simulink model "test_pi_av_formation_event_gazebodirected23a"  (R2023a)
settings: Solver=FixedStepAuto  StartTime=0.0  StopTime=inf  RelTol=1e-3
undefined symbols (not defined in the file or in its folder): angular, DiscIntNeverNeededParam, linear
libraries: ros2lib x28, simulink x8, robotcorelib x8
(part 2 of 4)

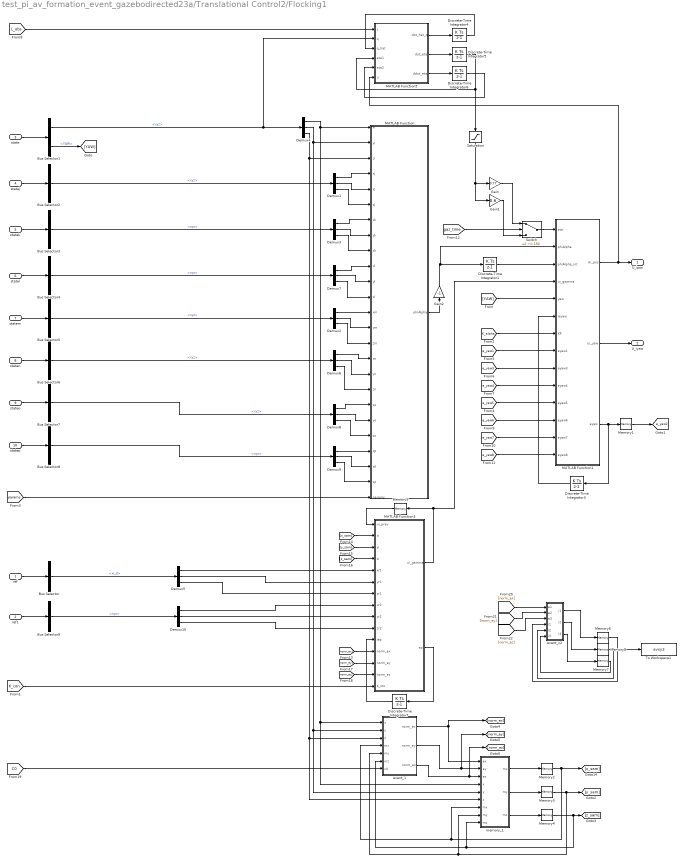
== system test_pi_av_formation_event_gazebodirected23a/Translational Control2/Flocking1 ==
  ref : Inport
  ref1 : Inport  Port=2
  state : Inport  Port=3
  statej : Inport  Port=4
  statek : Inport  Port=5
  statel : Inport  Port=6
  statem : Inport  Port=7
  staten : Inport  Port=8
  stateo : Inport  Port=9
  statep : Inport  Port=10
  Bus Selector : BusSelector  OutputSignals=xi_d
  Bus Selector1 : BusSelector  OutputSignals=xyz,YAW
  Bus Selector{2..9} (8 alike) : BusSelector  OutputSignals=xyz
  Demux{1..10} (10 alike) : Demux  Outputs=3
  Discrete-Time Integrator1 : DiscreteIntegrator  SampleTime=-1  LimitOutput=on  UpperSaturationLimit=2  LowerSaturationLimit=-2  ICPrevOutput=DiscIntNeverNeededParam  ICPrevScaledInput=DiscIntNeverNeededParam
  Discrete-Time Integrator3 : DiscreteIntegrator  SampleTime=-1  LimitOutput=on  UpperSaturationLimit=1  LowerSaturationLimit=-1  ICPrevOutput=DiscIntNeverNeededParam  ICPrevScaledInput=DiscIntNeverNeededParam
  Discrete-Time Integrator4 : DiscreteIntegrator  SampleTime=-1  LimitOutput=on  UpperSaturationLimit=5  LowerSaturationLimit=-5  ICPrevOutput=DiscIntNeverNeededParam  ICPrevScaledInput=DiscIntNeverNeededParam
  Discrete-Time Integrator5 : DiscreteIntegrator  SampleTime=-1  LimitOutput=on  UpperSaturationLimit=5  LowerSaturationLimit=-5  ICPrevOutput=DiscIntNeverNeededParam  ICPrevScaledInput=DiscIntNeverNeededParam
  Discrete-Time Integrator6 : DiscreteIntegrator  SampleTime=-1  LimitOutput=on  UpperSaturationLimit=0.2  LowerSaturationLimit=-0.2  ICPrevOutput=DiscIntNeverNeededParam  ICPrevScaledInput=DiscIntNeverNeededParam
  Discrete-Time Integrator7 : DiscreteIntegrator  SampleTime=-1  LimitOutput=on  UpperSaturationLimit=2  LowerSaturationLimit=-2  ICPrevOutput=DiscIntNeverNeededParam  ICPrevScaledInput=DiscIntNeverNeededParam
  Gain : Gain  Gain=0.77
  Gain1 : Gain  Gain=0.6
  Gain2 : Gain  Gain=-1
  MATLAB Function : MATLAB Function  TreatAsAtomicUnit=on
  MATLAB Function1 : MATLAB Function  TreatAsAtomicUnit=on
  MATLAB Function3 : MATLAB Function  TreatAsAtomicUnit=on
  MATLAB Function5 : MATLAB Function  TreatAsAtomicUnit=on
  Memory1 : Memory  InitialCondition=1
  Memory{2..4,6..8} (6 alike) : Memory
  Memory5 : Memory  InitialCondition=[0 0 0]'
  Saturation : Saturate  UpperLimit=1  LowerLimit=-1
  Switch : Switch  Threshold=150  SaturateOnIntegerOverflow=off  InputSameDT=off
  To Workspace1 : ToWorkspace  VariableName=evsy2  SampleTime=-1
  event_1 : MATLAB Function  TreatAsAtomicUnit=on
  event_x2 : MATLAB Function  TreatAsAtomicUnit=on
  memory_1 : MATLAB Function  TreatAsAtomicUnit=on
  U_ipos : Outport  VectorParamsAs1DForOutWhenUnconnected=off
  U_iyaw : Outport  Port=2  VectorParamsAs1DForOutWhenUnconnected=off
  tag scope: e_yaw2=global
  wires:
  state/1 -> Bus Selector1/1
  statej/1 -> Bus Selector2/1
  Bus Selector2/1 -> Demux1/1  "<xyz>"
  Demux1/1 -> MATLAB Function/4(xj)
  Demux1/2 -> MATLAB Function/5(yj)
  Discrete-Time Integrator1/1 -> MATLAB Function1/3(phiAlpha_int)
  statek/1 -> Bus Selector3/1
  Demux3/1 -> MATLAB Function/7(xk)
  Demux3/2 -> MATLAB Function/8(yk)
  Bus Selector3/1 -> Demux3/1  "<xyz>"
  MATLAB Function/1(phiAlpha) -> Gain2/1
  Demux3/3 -> MATLAB Function/9(zk)
  Demux1/3 -> MATLAB Function/6(zj)
  statel/1 -> Bus Selector4/1
  Demux7/1 -> MATLAB Function/10(xl)
  Demux7/2 -> MATLAB Function/11(yl)
  Demux7/3 -> MATLAB Function/12(zl)
  Bus Selector4/1 -> Demux7/1  "<xyz>"
  Bus Selector1/2 -> [YAW]  "<YAW>"
  [YAW] -> MATLAB Function1/5(yaw)
  MATLAB Function1/2(ui_yaw) -> U_iyaw/1
  MATLAB Function1/3(eyaw) -> Memory1/1, Discrete-Time Integrator3/1
  Discrete-Time Integrator3/1 -> MATLAB Function1/6(ieyaw)
  [K_alpha] -> MATLAB Function1/7(KP)
  [params] -> MATLAB Function/25(params)
  statem/1 -> Bus Selector5/1
  Bus Selector5/1 -> Demux2/1  "<xyz>"
  Demux2/1 -> MATLAB Function/13(xm)
  Demux2/2 -> MATLAB Function/14(ym)
  Demux2/3 -> MATLAB Function/15(zm)
  Memory1/1 -> [e_yaw2]
  [e_yaw1] -> MATLAB Function1/8(eyaw1)
  [e_yaw3] -> MATLAB Function1/9(eyaw3)
  [e_yaw4] -> MATLAB Function1/10(eyaw4)
  [e_yaw5] -> MATLAB Function1/11(eyaw5)
  Discrete-Time Integrator4/1 -> MATLAB Function5/3(q_hat)
  Discrete-Time Integrator5/1 -> Saturation/1, MATLAB Function5/4(eta1)
  [L_obs] -> MATLAB Function5/1(L)
  MATLAB Function5/1(dot_hat_q) -> Discrete-Time Integrator4/1
  MATLAB Function1/1(Ui_pos) -> MATLAB Function5/6(u), U_ipos/1
  Bus Selector1/1 -> MATLAB Function5/2(q), Demux4/1  "<xyz>"
  MATLAB Function5/2(dot_eta) -> Discrete-Time Integrator5/1
  Discrete-Time Integrator6/1 -> MATLAB Function5/5(eta2)
  MATLAB Function5/3(ddot_eta) -> Discrete-Time Integrator6/1
  staten/1 -> Bus Selector6/1
  Demux6/1 -> MATLAB Function/16(xn)
  Demux6/2 -> MATLAB Function/17(yn)
  Demux6/3 -> MATLAB Function/18(zn)
  Bus Selector6/1 -> Demux6/1  "<xyz>"
  [e_yaw6] -> MATLAB Function1/12(eyaw6)
  stateo/1 -> Bus Selector7/1
  Demux8/1 -> MATLAB Function/19(xo)
  Demux8/2 -> MATLAB Function/20(yo)
  Demux8/3 -> MATLAB Function/21(zo)
  Bus Selector7/1 -> Demux8/1  "<xyz>"
  [e_yaw7] -> MATLAB Function1/13(eyaw7)
  statep/1 -> Bus Selector8/1
  Demux9/1 -> MATLAB Function/22(xp)
  Demux9/2 -> MATLAB Function/23(yp)
  Demux9/3 -> MATLAB Function/24(zp)
  Bus Selector8/1 -> Demux9/1  "<xyz>"
  [e_yaw8] -> MATLAB Function1/14(eyaw8)
  Bus Selector/1 -> Demux5/1  "<xi_d>"
  Demux5/1 -> MATLAB Function3/5(xr1)
  ref/1 -> Bus Selector/1
  Demux10/1 -> MATLAB Function3/8(xr2)
  [K_con] -> MATLAB Function3/15(K_cts)
  Demux5/2 -> MATLAB Function3/6(yr1)
  ref1/1 -> Bus Selector9/1
  Demux10/3 -> MATLAB Function3/10(zr2)
  Demux10/2 -> MATLAB Function3/9(yr2)
  Demux5/3 -> MATLAB Function3/7(zr1)
  Bus Selector9/1 -> Demux10/1  "<xyz>"
  Saturation/1 -> Gain1/1, Gain/1
  Switch/1 -> MATLAB Function1/1(eta)
  [gaz_time] -> Switch/2
  Gain1/1 -> Switch/3
  Gain/1 -> Switch/1
  event_1/2(norm_ey) -> [norm_ey], memory_1/2(ey)
  Memory4/1 -> memory_1/9("mz "), event_1/6(mz), [z_sam]
  memory_1/2(my) -> Memory3/1
  memory_1/3(mz) -> Memory4/1
  Memory3/1 -> [y_sam], memory_1/8("my "), event_1/5(my)
  Demux4/1 -> event_1/1(x), memory_1/4(x), MATLAB Function/1(xi)
  event_1/3(norm_ez) -> [norm_ez], memory_1/3(ez)
  Demux4/3 -> event_1/3(z), memory_1/6(z), MATLAB Function/3(zi)
  MATLAB Function3/2(ep) -> Discrete-Time Integrator7/1
  Discrete-Time Integrator7/1 -> MATLAB Function3/11(iep)
  Demux4/2 -> event_1/2(y), memory_1/5(y), MATLAB Function/2(yi)
  event_1/1(norm_ex) -> [norm_ex], memory_1/1(ex)
  memory_1/1(mx) -> Memory2/1
  Memory2/1 -> memory_1/7("mx "), event_1/4(mx), [x_sam]
  Memory5/1 -> MATLAB Function3/1(ui_prev)
  MATLAB Function3/1(ui_gamma) -> MATLAB Function1/4(ui_gamma), Memory5/1
  [x_sam] -> MATLAB Function3/2(xi)
  [y_sam] -> MATLAB Function3/3(yi)
  [z_sam] -> MATLAB Function3/4(zi)
  [norm_ex] -> MATLAB Function3/12(norm_ex)
  [norm_ey] -> MATLAB Function3/13(norm_ey)
  [norm_ez] -> MATLAB Function3/14(norm_ez)
  [C0] -> event_1/7(c0)
  Gain2/1 -> Discrete-Time Integrator1/1, MATLAB Function1/2(phiAlpha)
  Memory7/1 -> event_x2/6("i3 ")
  [norm_ez] -> event_x2/3(e3)
  [norm_ex] -> event_x2/1(e1)
  event_x2/2(i2) -> Memory8/1
  Memory8/1 -> To Workspace1/1, event_x2/5("i2 ")
  event_x2/1(i1) -> Memory6/1
  Memory6/1 -> event_x2/4("i1 ")
  event_x2/3(i3) -> Memory7/1
  [norm_ey] -> event_x2/2(e2)

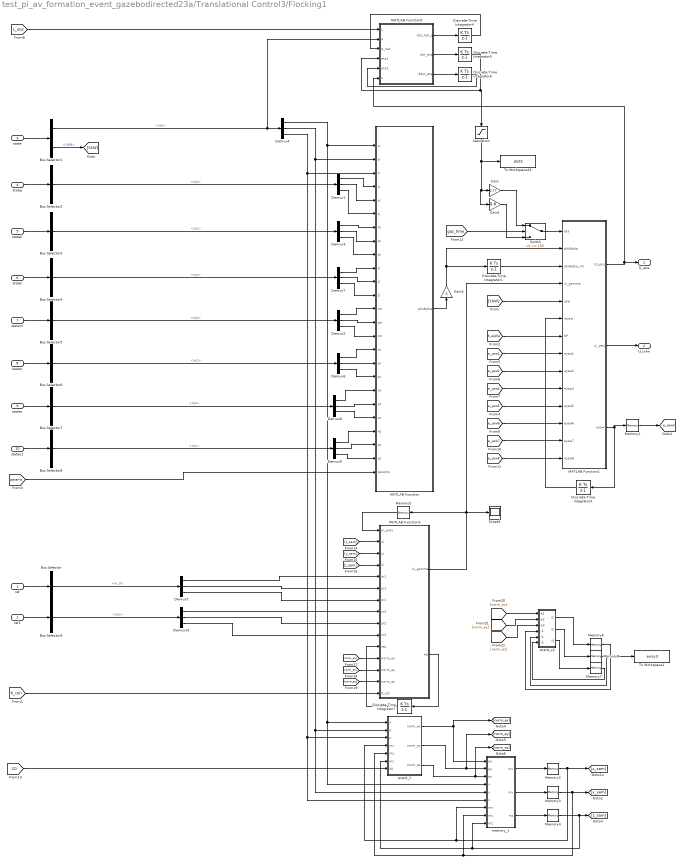
== system test_pi_av_formation_event_gazebodirected23a/Translational Control3/Flocking1 ==
  ref : Inport
  ref1 : Inport  Port=2
  state : Inport  Port=3
  statej : Inport  Port=4
  statek : Inport  Port=5
  statel : Inport  Port=6
  statem : Inport  Port=7
  staten : Inport  Port=8
  stateo : Inport  Port=9
  stateo1 : Inport  Port=10
  Bus Selector : BusSelector  OutputSignals=xi_d
  Bus Selector1 : BusSelector  OutputSignals=xyz,YAW
  Bus Selector{2..9} (8 alike) : BusSelector  OutputSignals=xyz
  Demux{1..10} (10 alike) : Demux  Outputs=3
  Discrete-Time Integrator1 : DiscreteIntegrator  SampleTime=-1  LimitOutput=on  UpperSaturationLimit=2  LowerSaturationLimit=-2  ICPrevOutput=DiscIntNeverNeededParam  ICPrevScaledInput=DiscIntNeverNeededParam
  Discrete-Time Integrator3 : DiscreteIntegrator  SampleTime=-1  LimitOutput=on  UpperSaturationLimit=1  LowerSaturationLimit=-1  ICPrevOutput=DiscIntNeverNeededParam  ICPrevScaledInput=DiscIntNeverNeededParam
  Discrete-Time Integrator4 : DiscreteIntegrator  SampleTime=-1  LimitOutput=on  UpperSaturationLimit=5  LowerSaturationLimit=-5  ICPrevOutput=DiscIntNeverNeededParam  ICPrevScaledInput=DiscIntNeverNeededParam
  Discrete-Time Integrator5 : DiscreteIntegrator  SampleTime=-1  LimitOutput=on  UpperSaturationLimit=2  LowerSaturationLimit=-2  ICPrevOutput=DiscIntNeverNeededParam  ICPrevScaledInput=DiscIntNeverNeededParam
  Discrete-Time Integrator6 : DiscreteIntegrator  SampleTime=-1  LimitOutput=on  UpperSaturationLimit=0.2  LowerSaturationLimit=-0.2  ICPrevOutput=DiscIntNeverNeededParam  ICPrevScaledInput=DiscIntNeverNeededParam
  Discrete-Time Integrator7 : DiscreteIntegrator  SampleTime=-1  LimitOutput=on  UpperSaturationLimit=2  LowerSaturationLimit=-2  ICPrevOutput=DiscIntNeverNeededParam  ICPrevScaledInput=DiscIntNeverNeededParam
  Gain : Gain  Gain=0.77
  Gain1 : Gain  Gain=0.6
  Gain2 : Gain  Gain=-1
  MATLAB Function : MATLAB Function  TreatAsAtomicUnit=on
  MATLAB Function1 : MATLAB Function  TreatAsAtomicUnit=on
  MATLAB Function3 : MATLAB Function  TreatAsAtomicUnit=on
  MATLAB Function5 : MATLAB Function  TreatAsAtomicUnit=on
  Memory1 : Memory  InitialCondition=1
  Memory{2..4,6..8} (6 alike) : Memory
  Memory5 : Memory  InitialCondition=[0 0 0]'
  Saturation : Saturate  UpperLimit=1  LowerLimit=-1
  Scope1 : Scope
  Switch : Switch  Threshold=150  SaturateOnIntegerOverflow=off  InputSameDT=off
  To Workspace1 : ToWorkspace  VariableName=evsy3  SampleTime=-1
  To Workspace24 : ToWorkspace  VariableName=dist3  SampleTime=-1
  event_1 : MATLAB Function  TreatAsAtomicUnit=on
  event_x2 : MATLAB Function  TreatAsAtomicUnit=on
  memory_1 : MATLAB Function  TreatAsAtomicUnit=on
  U_ipos : Outport  VectorParamsAs1DForOutWhenUnconnected=off
  U_iyaw : Outport  Port=2  VectorParamsAs1DForOutWhenUnconnected=off
  tag scope: e_yaw3=global
  wires:
  state/1 -> Bus Selector1/1
  statej/1 -> Bus Selector2/1
  Bus Selector2/1 -> Demux1/1  "<xyz>"
  Demux1/1 -> MATLAB Function/4(xj)
  Demux1/2 -> MATLAB Function/5(yj)
  Discrete-Time Integrator1/1 -> MATLAB Function1/3(phiAlpha_int)
  statek/1 -> Bus Selector3/1
  Demux3/1 -> MATLAB Function/7(xk)
  Demux3/2 -> MATLAB Function/8(yk)
  Bus Selector3/1 -> Demux3/1  "<xyz>"
  MATLAB Function/1(phiAlpha) -> Gain2/1
  Demux3/3 -> MATLAB Function/9(zk)
  Demux1/3 -> MATLAB Function/6(zj)
  statel/1 -> Bus Selector4/1
  Demux7/1 -> MATLAB Function/10(xl)
  Demux7/2 -> MATLAB Function/11(yl)
  Demux7/3 -> MATLAB Function/12(zl)
  Bus Selector4/1 -> Demux7/1  "<xyz>"
  Bus Selector1/2 -> [YAW]  "<YAW>"
  [YAW] -> MATLAB Function1/5(yaw)
  MATLAB Function1/2(ui_yaw) -> U_iyaw/1
  MATLAB Function1/3(eyaw) -> Memory1/1, Discrete-Time Integrator3/1
  Discrete-Time Integrator3/1 -> MATLAB Function1/6(ieyaw)
  [K_alpha] -> MATLAB Function1/7(KP)
  [params] -> MATLAB Function/25(params)
  statem/1 -> Bus Selector5/1
  Bus Selector5/1 -> Demux2/1  "<xyz>"
  Demux2/1 -> MATLAB Function/13(xm)
  Demux2/2 -> MATLAB Function/14(ym)
  Demux2/3 -> MATLAB Function/15(zm)
  Memory1/1 -> [e_yaw3]
  [e_yaw1] -> MATLAB Function1/8(eyaw1)
  [e_yaw2] -> MATLAB Function1/9(eyaw2)
  [e_yaw4] -> MATLAB Function1/10(eyaw4)
  [e_yaw5] -> MATLAB Function1/11(eyaw5)
  Discrete-Time Integrator4/1 -> MATLAB Function5/3(q_hat)
  Discrete-Time Integrator5/1 -> Saturation/1, MATLAB Function5/4(eta1)
  [L_obs] -> MATLAB Function5/1(L)
  MATLAB Function5/1(dot_hat_q) -> Discrete-Time Integrator4/1
  MATLAB Function1/1(Ui_pos) -> MATLAB Function5/6(u), U_ipos/1
  Bus Selector1/1 -> MATLAB Function5/2(q), Demux4/1  "<xyz>"
  MATLAB Function5/2(dot_eta) -> Discrete-Time Integrator5/1
  Discrete-Time Integrator6/1 -> MATLAB Function5/5(eta2)
  MATLAB Function5/3(ddot_eta) -> Discrete-Time Integrator6/1
  staten/1 -> Bus Selector6/1
  Demux6/1 -> MATLAB Function/16(xn)
  Demux6/2 -> MATLAB Function/17(yn)
  Demux6/3 -> MATLAB Function/18(zn)
  Bus Selector6/1 -> Demux6/1  "<xyz>"
  [e_yaw6] -> MATLAB Function1/12(eyaw6)
  [e_yaw7] -> MATLAB Function1/13(eyaw7)
  stateo/1 -> Bus Selector7/1
  Demux8/1 -> MATLAB Function/19(xo)
  Demux8/2 -> MATLAB Function/20(yo)
  Demux8/3 -> MATLAB Function/21(zo)
  Bus Selector7/1 -> Demux8/1  "<xyz>"
  stateo1/1 -> Bus Selector8/1
  Demux9/1 -> MATLAB Function/22(xp)
  Demux9/2 -> MATLAB Function/23(yp)
  Demux9/3 -> MATLAB Function/24(zp)
  Bus Selector8/1 -> Demux9/1  "<xyz>"
  [e_yaw8] -> MATLAB Function1/14(eyaw8)
  Bus Selector/1 -> Demux5/1  "<xi_d>"
  ref/1 -> Bus Selector/1
  ref1/1 -> Bus Selector9/1
  Bus Selector9/1 -> Demux10/1  "<xyz>"
  Switch/1 -> MATLAB Function1/1(eta)
  [gaz_time] -> Switch/2
  Gain1/1 -> Switch/3
  Gain/1 -> Switch/1
  Saturation/1 -> To Workspace24/1, Gain1/1, Gain/1
  Memory4/1 -> memory_1/9("mz "), event_1/6(mz), [z_sam]
  memory_1/2(my) -> Memory3/1
  memory_1/3(mz) -> Memory4/1
  Memory3/1 -> [y_sam], memory_1/8("my "), event_1/5(my)
  Demux4/1 -> memory_1/4(x), event_1/1(x), MATLAB Function/1(xi)
  event_1/3(norm_ez) -> [norm_ez], memory_1/3(ez)
  event_1/1(norm_ex) -> [norm_ex], memory_1/1(ex)
  MATLAB Function3/1(ui_gamma) -> MATLAB Function1/4(ui_gamma), Scope1/1, Memory5/1
  event_1/2(norm_ey) -> [norm_ey], memory_1/2(ey)
  Demux4/3 -> memory_1/6(z), event_1/3(z), MATLAB Function/3(zi)
  MATLAB Function3/2(ep) -> Discrete-Time Integrator7/1
  memory_1/1(mx) -> Memory2/1
  Discrete-Time Integrator7/1 -> MATLAB Function3/11(iep)
  Demux4/2 -> memory_1/5(y), event_1/2(y), MATLAB Function/2(yi)
  Memory2/1 -> memory_1/7("mx "), event_1/4(mx), [x_sam]
  Memory5/1 -> MATLAB Function3/1(ui_prev)
  [K_con] -> MATLAB Function3/15(K_cts)
  Demux5/1 -> MATLAB Function3/5(xr1)
  Demux5/2 -> MATLAB Function3/6(yr1)
  Demux5/3 -> MATLAB Function3/7(zr1)
  Demux10/1 -> MATLAB Function3/8(xr2)
  Demux10/2 -> MATLAB Function3/9(yr2)
  Demux10/3 -> MATLAB Function3/10(zr2)
  [y_sam] -> MATLAB Function3/3(yi)
  [x_sam] -> MATLAB Function3/2(xi)
  [z_sam] -> MATLAB Function3/4(zi)
  [norm_ez] -> MATLAB Function3/14(norm_ez)
  [norm_ey] -> MATLAB Function3/13(norm_ey)
  [norm_ex] -> MATLAB Function3/12(norm_ex)
  [C0] -> event_1/7(c0)
  Gain2/1 -> MATLAB Function1/2(phiAlpha), Discrete-Time Integrator1/1
  Memory7/1 -> event_x2/6("i3 ")
  [norm_ez] -> event_x2/3(e3)
  [norm_ex] -> event_x2/1(e1)
  event_x2/2(i2) -> Memory8/1
  Memory8/1 -> To Workspace1/1, event_x2/5("i2 ")
  event_x2/1(i1) -> Memory6/1
  Memory6/1 -> event_x2/4("i1 ")
  event_x2/3(i3) -> Memory7/1
  [norm_ey] -> event_x2/2(e2)

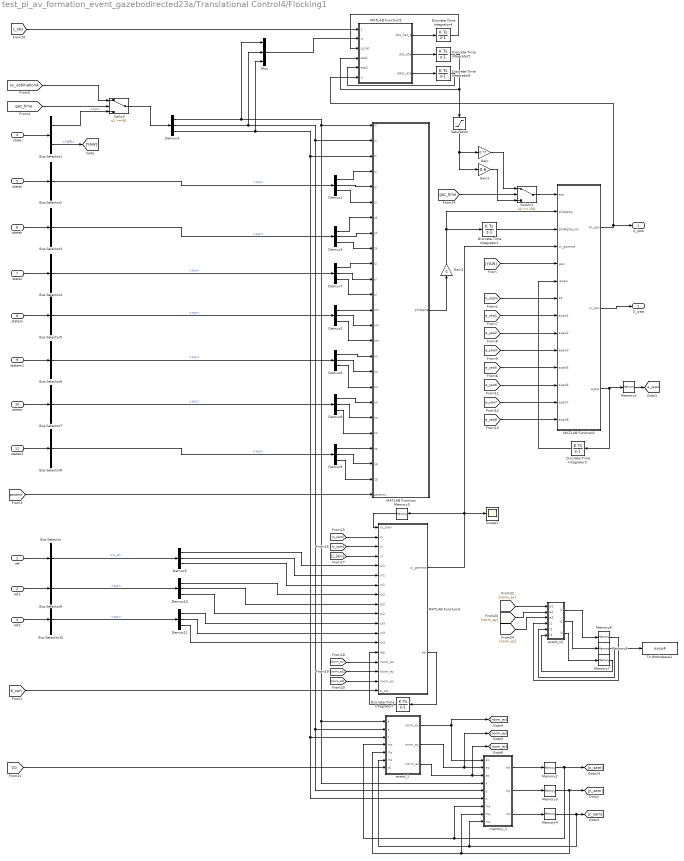
== system test_pi_av_formation_event_gazebodirected23a/Translational Control4/Flocking1 ==
  ref : Inport
  ref1 : Inport  Port=2
  ref2 : Inport  Port=3
  state : Inport  Port=4
  statej : Inport  Port=5
  statek : Inport  Port=6
  statel : Inport  Port=7
  statem : Inport  Port=8
  statem1 : Inport  Port=9
  stateo : Inport  Port=10
  stateo1 : Inport  Port=11
  Bus Selector : BusSelector  OutputSignals=xi_d
  Bus Selector1 : BusSelector  OutputSignals=xyz,YAW
  Bus Selector{2..10} (9 alike) : BusSelector  OutputSignals=xyz
  Demux{1..11} (11 alike) : Demux  Outputs=3
  Discrete-Time Integrator1 : DiscreteIntegrator  SampleTime=-1  LimitOutput=on  UpperSaturationLimit=2  LowerSaturationLimit=-2  ICPrevOutput=DiscIntNeverNeededParam  ICPrevScaledInput=DiscIntNeverNeededParam
  Discrete-Time Integrator3 : DiscreteIntegrator  SampleTime=-1  LimitOutput=on  UpperSaturationLimit=1  LowerSaturationLimit=-1  ICPrevOutput=DiscIntNeverNeededParam  ICPrevScaledInput=DiscIntNeverNeededParam
  Discrete-Time Integrator4 : DiscreteIntegrator  SampleTime=-1  LimitOutput=on  UpperSaturationLimit=5  LowerSaturationLimit=-5  ICPrevOutput=DiscIntNeverNeededParam  ICPrevScaledInput=DiscIntNeverNeededParam
  Discrete-Time Integrator5 : DiscreteIntegrator  SampleTime=-1  LimitOutput=on  UpperSaturationLimit=5  LowerSaturationLimit=-5  ICPrevOutput=DiscIntNeverNeededParam  ICPrevScaledInput=DiscIntNeverNeededParam
  Discrete-Time Integrator6 : DiscreteIntegrator  SampleTime=-1  LimitOutput=on  UpperSaturationLimit=0.2  LowerSaturationLimit=-0.2  ICPrevOutput=DiscIntNeverNeededParam  ICPrevScaledInput=DiscIntNeverNeededParam
  Discrete-Time Integrator7 : DiscreteIntegrator  SampleTime=-1  LimitOutput=on  UpperSaturationLimit=2  LowerSaturationLimit=-2  ICPrevOutput=DiscIntNeverNeededParam  ICPrevScaledInput=DiscIntNeverNeededParam
  Gain : Gain  Gain=0.77
  Gain1 : Gain  Gain=0.6
  Gain2 : Gain  Gain=-1
  MATLAB Function : MATLAB Function  TreatAsAtomicUnit=on
  MATLAB Function1 : MATLAB Function  TreatAsAtomicUnit=on
  MATLAB Function3 : MATLAB Function  TreatAsAtomicUnit=on
  MATLAB Function5 : MATLAB Function  TreatAsAtomicUnit=on
  Memory1 : Memory  InitialCondition=1
  Memory{2..4,6..8} (6 alike) : Memory
  Memory5 : Memory  InitialCondition=[0 0 0]'
  Mux : Mux  Inputs=3
  Saturation : Saturate  UpperLimit=1  LowerLimit=-1
  Scope1 : Scope
  Switch : Switch  Threshold=60  SaturateOnIntegerOverflow=off  InputSameDT=off
  Switch1 : Switch  Threshold=150  SaturateOnIntegerOverflow=off  InputSameDT=off
  To Workspace1 : ToWorkspace  VariableName=evsy4  SampleTime=-1
  event_1 : MATLAB Function  TreatAsAtomicUnit=on
  event_x2 : MATLAB Function  TreatAsAtomicUnit=on
  memory_1 : MATLAB Function  TreatAsAtomicUnit=on
  U_ipos : Outport  VectorParamsAs1DForOutWhenUnconnected=off
  U_iyaw : Outport  Port=2  VectorParamsAs1DForOutWhenUnconnected=off
  tag scope: e_yaw4=global
  wires:
  ref/1 -> Bus Selector/1
  state/1 -> Bus Selector1/1
  Bus Selector/1 -> Demux5/1  "<xi_d>"
  statej/1 -> Bus Selector2/1
  Bus Selector2/1 -> Demux1/1  "<xyz>"
  Demux1/1 -> MATLAB Function/4(xj)
  Demux1/2 -> MATLAB Function/5(yj)
  Discrete-Time Integrator1/1 -> MATLAB Function1/3(phiAlpha_int)
  statek/1 -> Bus Selector3/1
  Demux3/1 -> MATLAB Function/7(xk)
  Demux3/2 -> MATLAB Function/8(yk)
  Bus Selector3/1 -> Demux3/1  "<xyz>"
  MATLAB Function/1(phiAlpha) -> Gain2/1
  Demux3/3 -> MATLAB Function/9(zk)
  Demux1/3 -> MATLAB Function/6(zj)
  statel/1 -> Bus Selector4/1
  Demux7/1 -> MATLAB Function/10(xl)
  Demux7/2 -> MATLAB Function/11(yl)
  Demux7/3 -> MATLAB Function/12(zl)
  Bus Selector4/1 -> Demux7/1  "<xyz>"
  Bus Selector1/2 -> [YAW]  "<YAW>"
  [YAW] -> MATLAB Function1/5(yaw)
  MATLAB Function1/2(ui_yaw) -> U_iyaw/1
  [K_con] -> MATLAB Function3/18(K_cts)
  MATLAB Function1/3(eyaw) -> Memory1/1, Discrete-Time Integrator3/1
  Discrete-Time Integrator3/1 -> MATLAB Function1/6(ieyaw)
  [K_alpha] -> MATLAB Function1/7(KP)
  [params] -> MATLAB Function/25(params)
  statem/1 -> Bus Selector5/1
  Bus Selector5/1 -> Demux2/1  "<xyz>"
  Demux2/1 -> MATLAB Function/13(xm)
  Demux2/2 -> MATLAB Function/14(ym)
  Demux2/3 -> MATLAB Function/15(zm)
  [gaz_time] -> Switch/2
  [xy_estimation4] -> Switch/1
  [e_yaw1] -> MATLAB Function1/8(eyaw1)
  [e_yaw2] -> MATLAB Function1/9(eyaw2)
  [e_yaw3] -> MATLAB Function1/10(eyaw3)
  [e_yaw5] -> MATLAB Function1/11(eyaw5)
  Memory1/1 -> [e_yaw4]
  Mux/1 -> MATLAB Function5/2(q)
  MATLAB Function5/1(dot_hat_q) -> Discrete-Time Integrator4/1
  Discrete-Time Integrator6/1 -> MATLAB Function5/5(eta2)
  MATLAB Function5/3(ddot_eta) -> Discrete-Time Integrator6/1
  Discrete-Time Integrator5/1 -> Saturation/1, MATLAB Function5/4(eta1)
  MATLAB Function5/2(dot_eta) -> Discrete-Time Integrator5/1
  Discrete-Time Integrator4/1 -> MATLAB Function5/3(q_hat)
  [L_obs] -> MATLAB Function5/1(L)
  MATLAB Function1/1(Ui_pos) -> MATLAB Function5/6(u), U_ipos/1
  statem1/1 -> Bus Selector6/1
  Demux6/1 -> MATLAB Function/16(xn)
  Demux6/2 -> MATLAB Function/17(yn)
  Demux6/3 -> MATLAB Function/18(zn)
  Bus Selector6/1 -> Demux6/1  "<xyz>"
  Bus Selector1/1 -> Switch/3  "<xyz>"
  Switch/1 -> Demux4/1
  stateo/1 -> Bus Selector7/1
  Demux8/1 -> MATLAB Function/19(xo)
  Demux8/2 -> MATLAB Function/20(yo)
  Demux8/3 -> MATLAB Function/21(zo)
  Bus Selector7/1 -> Demux8/1  "<xyz>"
  [e_yaw6] -> MATLAB Function1/12(eyaw6)
  [e_yaw7] -> MATLAB Function1/13(eyaw7)
  stateo1/1 -> Bus Selector8/1
  Demux9/1 -> MATLAB Function/22(xp)
  Demux9/2 -> MATLAB Function/23(yp)
  Demux9/3 -> MATLAB Function/24(zp)
  Bus Selector8/1 -> Demux9/1  "<xyz>"
  [e_yaw8] -> MATLAB Function1/14(eyaw8)
  Bus Selector9/1 -> Demux10/1  "<xyz>"
  ref1/1 -> Bus Selector9/1
  Switch1/1 -> MATLAB Function1/1(eta)
  Gain/1 -> Switch1/1
  Gain1/1 -> Switch1/3
  [gaz_time] -> Switch1/2
  Saturation/1 -> Gain1/1, Gain/1
  ref2/1 -> Bus Selector10/1
  Bus Selector10/1 -> Demux11/1  "<xyz>"
  event_1/2(norm_ey) -> [norm_ey], memory_1/2(ey)
  MATLAB Function3/1(ui_gamma) -> MATLAB Function1/4(ui_gamma), Scope1/1, Memory5/1
  Memory4/1 -> memory_1/9("mz "), event_1/6(mz), [z_sam]
  memory_1/2(my) -> Memory3/1
  memory_1/3(mz) -> Memory4/1
  Memory3/1 -> [y_sam], memory_1/8("my "), event_1/5(my)
  Demux4/1 -> Mux/1, event_1/1(x), memory_1/4(x), MATLAB Function/1(xi)
  event_1/3(norm_ez) -> [norm_ez], memory_1/3(ez)
  Demux4/3 -> Mux/3, event_1/3(z), memory_1/6(z), MATLAB Function/3(zi)
  MATLAB Function3/2(ep) -> Discrete-Time Integrator7/1
  memory_1/1(mx) -> Memory2/1
  Discrete-Time Integrator7/1 -> MATLAB Function3/14(iep)
  Demux4/2 -> Mux/2, event_1/2(y), memory_1/5(y), MATLAB Function/2(yi)
  event_1/1(norm_ex) -> [norm_ex], memory_1/1(ex)
  Memory2/1 -> memory_1/7("mx "), event_1/4(mx), [x_sam]
  Memory5/1 -> MATLAB Function3/1(ui_prev)
  [x_sam] -> MATLAB Function3/2(xi)
  [y_sam] -> MATLAB Function3/3(yi)
  [z_sam] -> MATLAB Function3/4(zi)
  [norm_ex] -> MATLAB Function3/15(norm_ex)
  [norm_ey] -> MATLAB Function3/16(norm_ey)
  [norm_ez] -> MATLAB Function3/17(norm_ez)
  Demux5/1 -> MATLAB Function3/5(xr1)
  Demux5/2 -> MATLAB Function3/6(yr1)
  Demux5/3 -> MATLAB Function3/7(zr1)
  Demux10/1 -> MATLAB Function3/8(xr2)
  Demux10/2 -> MATLAB Function3/9(yr2)
  Demux10/3 -> MATLAB Function3/10(zr2)
  Demux11/1 -> MATLAB Function3/11(xr3)
  Demux11/2 -> MATLAB Function3/12(yr3)
  Demux11/3 -> MATLAB Function3/13(zr3)
  [C0] -> event_1/7(c0)
  Gain2/1 -> MATLAB Function1/2(phiAlpha), Discrete-Time Integrator1/1
  Memory7/1 -> event_x2/6("i3 ")
  [norm_ez] -> event_x2/3(e3)
  [norm_ex] -> event_x2/1(e1)
  event_x2/2(i2) -> Memory8/1
  Memory8/1 -> To Workspace1/1, event_x2/5("i2 ")
  event_x2/1(i1) -> Memory6/1
  Memory6/1 -> event_x2/4("i1 ")
  event_x2/3(i3) -> Memory7/1
  [norm_ey] -> event_x2/2(e2)

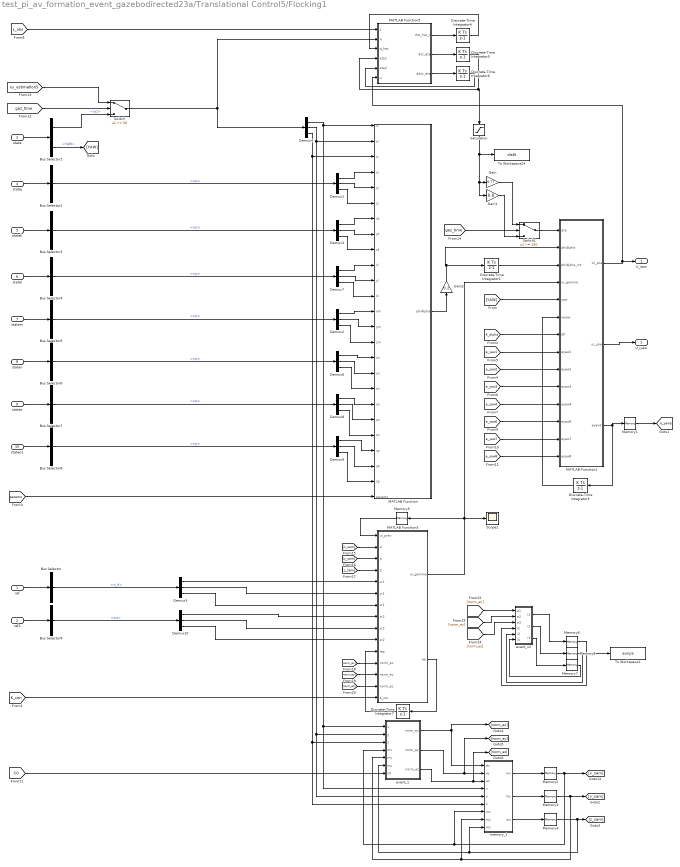
== system test_pi_av_formation_event_gazebodirected23a/Translational Control5/Flocking1 ==
  ref : Inport
  ref1 : Inport  Port=2
  state : Inport  Port=3
  statej : Inport  Port=4
  statek : Inport  Port=5
  statel : Inport  Port=6
  statem : Inport  Port=7
  staten : Inport  Port=8
  stateo : Inport  Port=9
  stateo1 : Inport  Port=10
  Bus Selector : BusSelector  OutputSignals=xi_d
  Bus Selector1 : BusSelector  OutputSignals=xyz,YAW
  Bus Selector{2..9} (8 alike) : BusSelector  OutputSignals=xyz
  Demux{1..10} (10 alike) : Demux  Outputs=3
  Discrete-Time Integrator1 : DiscreteIntegrator  SampleTime=-1  LimitOutput=on  UpperSaturationLimit=2  LowerSaturationLimit=-2  ICPrevOutput=DiscIntNeverNeededParam  ICPrevScaledInput=DiscIntNeverNeededParam
  Discrete-Time Integrator3 : DiscreteIntegrator  SampleTime=-1  LimitOutput=on  UpperSaturationLimit=1  LowerSaturationLimit=-1  ICPrevOutput=DiscIntNeverNeededParam  ICPrevScaledInput=DiscIntNeverNeededParam
  Discrete-Time Integrator4 : DiscreteIntegrator  SampleTime=-1  LimitOutput=on  UpperSaturationLimit=5  LowerSaturationLimit=-5  ICPrevOutput=DiscIntNeverNeededParam  ICPrevScaledInput=DiscIntNeverNeededParam
  Discrete-Time Integrator5 : DiscreteIntegrator  SampleTime=-1  LimitOutput=on  UpperSaturationLimit=5  LowerSaturationLimit=-5  ICPrevOutput=DiscIntNeverNeededParam  ICPrevScaledInput=DiscIntNeverNeededParam
  Discrete-Time Integrator6 : DiscreteIntegrator  SampleTime=-1  LimitOutput=on  UpperSaturationLimit=0.4  LowerSaturationLimit=-0.4  ICPrevOutput=DiscIntNeverNeededParam  ICPrevScaledInput=DiscIntNeverNeededParam
  Discrete-Time Integrator7 : DiscreteIntegrator  SampleTime=-1  LimitOutput=on  UpperSaturationLimit=2  LowerSaturationLimit=-2  ICPrevOutput=DiscIntNeverNeededParam  ICPrevScaledInput=DiscIntNeverNeededParam
  Gain : Gain  Gain=0.77
  Gain1 : Gain  Gain=0.6
  Gain2 : Gain  Gain=0.2
  MATLAB Function : MATLAB Function  TreatAsAtomicUnit=on
  MATLAB Function1 : MATLAB Function  TreatAsAtomicUnit=on
  MATLAB Function3 : MATLAB Function  TreatAsAtomicUnit=on
  MATLAB Function5 : MATLAB Function  TreatAsAtomicUnit=on
  Memory1 : Memory  InitialCondition=1
  Memory{2..4,6..8} (6 alike) : Memory
  Memory5 : Memory  InitialCondition=[0 0 0]'
  Saturation : Saturate  UpperLimit=1  LowerLimit=-1
  Scope1 : Scope
  Switch : Switch  Threshold=50  SaturateOnIntegerOverflow=off  InputSameDT=off
  Switch1 : Switch  Threshold=150  SaturateOnIntegerOverflow=off  InputSameDT=off
  To Workspace1 : ToWorkspace  VariableName=evsy5  SampleTime=-1
  To Workspace24 : ToWorkspace  VariableName=dist5  SampleTime=-1
  event_1 : MATLAB Function  TreatAsAtomicUnit=on
  event_x2 : MATLAB Function  TreatAsAtomicUnit=on
  memory_1 : MATLAB Function  TreatAsAtomicUnit=on
  U_ipos : Outport  VectorParamsAs1DForOutWhenUnconnected=off
  U_iyaw : Outport  Port=2  VectorParamsAs1DForOutWhenUnconnected=off
  tag scope: e_yaw5=global
  wires:
  ref/1 -> Bus Selector/1
  state/1 -> Bus Selector1/1
  Bus Selector/1 -> Demux5/1  "<xi_d>"
  statej/1 -> Bus Selector2/1
  Bus Selector2/1 -> Demux1/1  "<xyz>"
  Demux1/1 -> MATLAB Function/4(xj)
  Demux1/2 -> MATLAB Function/5(yj)
  Discrete-Time Integrator1/1 -> MATLAB Function1/3(phiAlpha_int)
  statek/1 -> Bus Selector3/1
  Demux3/1 -> MATLAB Function/7(xk)
  Demux3/2 -> MATLAB Function/8(yk)
  Bus Selector3/1 -> Demux3/1  "<xyz>"
  MATLAB Function/1(phiAlpha) -> Gain2/1
  Demux3/3 -> MATLAB Function/9(zk)
  Demux1/3 -> MATLAB Function/6(zj)
  statel/1 -> Bus Selector4/1
  Demux7/1 -> MATLAB Function/10(xl)
  Demux7/2 -> MATLAB Function/11(yl)
  Demux7/3 -> MATLAB Function/12(zl)
  Bus Selector4/1 -> Demux7/1  "<xyz>"
  Bus Selector1/2 -> [YAW]  "<YAW>"
  [YAW] -> MATLAB Function1/5(yaw)
  MATLAB Function1/2(ui_yaw) -> U_iyaw/1
  MATLAB Function1/3(eyaw2) -> Memory1/1, Discrete-Time Integrator3/1
  Discrete-Time Integrator3/1 -> MATLAB Function1/6(ieyaw)
  [K_alpha] -> MATLAB Function1/7(KP)
  [params] -> MATLAB Function/25(params)
  statem/1 -> Bus Selector5/1
  Bus Selector5/1 -> Demux2/1  "<xyz>"
  Demux2/1 -> MATLAB Function/13(xm)
  Demux2/2 -> MATLAB Function/14(ym)
  Demux2/3 -> MATLAB Function/15(zm)
  Memory1/1 -> [e_yaw5]
  [e_yaw1] -> MATLAB Function1/8(eyaw1)
  [e_yaw3] -> MATLAB Function1/10(eyaw3)
  [e_yaw4] -> MATLAB Function1/11(eyaw4)
  [e_yaw2] -> MATLAB Function1/9("eyaw2 ")
  Discrete-Time Integrator4/1 -> MATLAB Function5/3(q_hat)
  Discrete-Time Integrator5/1 -> Saturation/1, MATLAB Function5/4(eta1)
  [L_obs] -> MATLAB Function5/1(L)
  MATLAB Function5/1(dot_hat_q) -> Discrete-Time Integrator4/1
  MATLAB Function1/1(Ui_pos) -> MATLAB Function5/6(u), U_ipos/1
  MATLAB Function5/2(dot_eta) -> Discrete-Time Integrator5/1
  Discrete-Time Integrator6/1 -> MATLAB Function5/5(eta2)
  MATLAB Function5/3(ddot_eta) -> Discrete-Time Integrator6/1
  staten/1 -> Bus Selector6/1
  Demux6/1 -> MATLAB Function/16(xn)
  Demux6/2 -> MATLAB Function/17(yn)
  Demux6/3 -> MATLAB Function/18(zn)
  Bus Selector6/1 -> Demux6/1  "<xyz>"
  [e_yaw6] -> MATLAB Function1/12(eyaw6)
  stateo/1 -> Bus Selector7/1
  Demux8/1 -> MATLAB Function/19(xo)
  Demux8/2 -> MATLAB Function/20(yo)
  Demux8/3 -> MATLAB Function/21(zo)
  Bus Selector7/1 -> Demux8/1  "<xyz>"
  [e_yaw7] -> MATLAB Function1/13(eyaw7)
  stateo1/1 -> Bus Selector8/1
  Demux9/1 -> MATLAB Function/22(xp)
  Demux9/2 -> MATLAB Function/23(yp)
  Demux9/3 -> MATLAB Function/24(zp)
  Bus Selector8/1 -> Demux9/1  "<xyz>"
  [e_yaw8] -> MATLAB Function1/14(eyaw8)
  Switch/1 -> MATLAB Function5/2(q), Demux4/1
  Bus Selector1/1 -> Switch/3  "<xyz>"
  [xy_estimation5] -> Switch/1
  [gaz_time] -> Switch/2
  Bus Selector9/1 -> Demux10/1  "<xyz>"
  ref1/1 -> Bus Selector9/1
  Saturation/1 -> To Workspace24/1, Gain1/1, Gain/1
  Switch1/1 -> MATLAB Function1/1(eta)
  Gain1/1 -> Switch1/3
  Gain/1 -> Switch1/1
  [gaz_time] -> Switch1/2
  MATLAB Function3/1(ui_gamma) -> MATLAB Function1/4(ui_gamma), Scope1/1, Memory5/1
  event_1/1(norm_ex) -> [norm_ex], memory_1/1(ex)
  Demux4/1 -> memory_1/4(x), event_1/1(x), MATLAB Function/1(xi)
  event_1/3(norm_ez) -> [norm_ez], memory_1/3(ez)
  Demux4/2 -> memory_1/5(y), event_1/2(y), MATLAB Function/2(yi)
  Demux4/3 -> memory_1/6(z), event_1/3(z), MATLAB Function/3(zi)
  Memory4/1 -> memory_1/9("mz "), event_1/6(mz), [z_sam]
  Memory2/1 -> memory_1/7("mx "), event_1/4(mx), [x_sam]
  [y_sam] -> MATLAB Function3/3(yi)
  memory_1/3(mz) -> Memory4/1
  Memory5/1 -> MATLAB Function3/1(ui_prev)
  Memory3/1 -> [y_sam], memory_1/8("my "), event_1/5(my)
  [norm_ey] -> MATLAB Function3/13(norm_ey)
  [x_sam] -> MATLAB Function3/2(xi)
  event_1/2(norm_ey) -> [norm_ey], memory_1/2(ey)
  MATLAB Function3/2(ep) -> Discrete-Time Integrator7/1
  memory_1/1(mx) -> Memory2/1
  Discrete-Time Integrator7/1 -> MATLAB Function3/11(iep)
  [z_sam] -> MATLAB Function3/4(zi)
  memory_1/2(my) -> Memory3/1
  [norm_ez] -> MATLAB Function3/14(norm_ez)
  [norm_ex] -> MATLAB Function3/12(norm_ex)
  Demux5/1 -> MATLAB Function3/5(xr1)
  Demux5/2 -> MATLAB Function3/6(yr1)
  Demux5/3 -> MATLAB Function3/7(zr1)
  Demux10/1 -> MATLAB Function3/8(xr2)
  Demux10/2 -> MATLAB Function3/9(yr2)
  Demux10/3 -> MATLAB Function3/10(zr2)
  [K_con] -> MATLAB Function3/15(K_cts)
  [C0] -> event_1/7(c0)
  Gain2/1 -> MATLAB Function1/2(phiAlpha), Discrete-Time Integrator1/1
  Memory7/1 -> event_x2/6("i3 ")
  [norm_ez] -> event_x2/3(e3)
  [norm_ex] -> event_x2/1(e1)
  event_x2/2(i2) -> Memory8/1
  Memory8/1 -> To Workspace1/1, event_x2/5("i2 ")
  event_x2/1(i1) -> Memory6/1
  Memory6/1 -> event_x2/4("i1 ")
  event_x2/3(i3) -> Memory7/1
  [norm_ey] -> event_x2/2(e2)

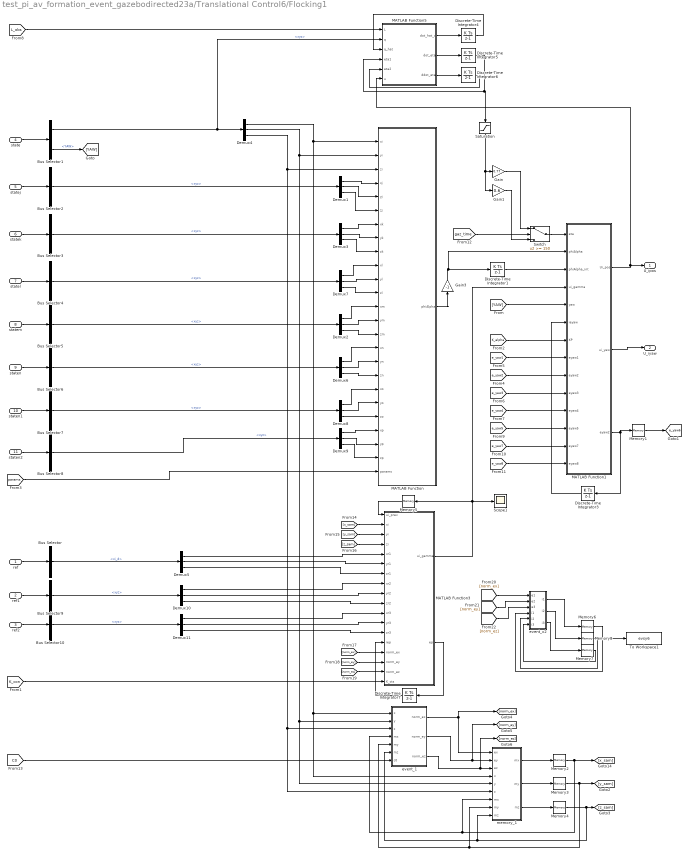
== system test_pi_av_formation_event_gazebodirected23a/Translational Control6/Flocking1 ==
  ref : Inport
  ref1 : Inport  Port=2
  ref2 : Inport  Port=3
  state : Inport  Port=4
  statej : Inport  Port=5
  statek : Inport  Port=6
  statel : Inport  Port=7
  statem : Inport  Port=8
  staten : Inport  Port=9
  staten1 : Inport  Port=10
  staten2 : Inport  Port=11
  Bus Selector : BusSelector  OutputSignals=xi_d
  Bus Selector1 : BusSelector  OutputSignals=xyz,YAW
  Bus Selector{2..10} (9 alike) : BusSelector  OutputSignals=xyz
  Demux{1..11} (11 alike) : Demux  Outputs=3
  Discrete-Time Integrator1 : DiscreteIntegrator  SampleTime=-1  LimitOutput=on  UpperSaturationLimit=2  LowerSaturationLimit=-2  ICPrevOutput=DiscIntNeverNeededParam  ICPrevScaledInput=DiscIntNeverNeededParam
  Discrete-Time Integrator3 : DiscreteIntegrator  SampleTime=-1  LimitOutput=on  UpperSaturationLimit=1  LowerSaturationLimit=-1  ICPrevOutput=DiscIntNeverNeededParam  ICPrevScaledInput=DiscIntNeverNeededParam
  Discrete-Time Integrator4 : DiscreteIntegrator  SampleTime=-1  LimitOutput=on  UpperSaturationLimit=5  LowerSaturationLimit=-5  ICPrevOutput=DiscIntNeverNeededParam  ICPrevScaledInput=DiscIntNeverNeededParam
  Discrete-Time Integrator5 : DiscreteIntegrator  SampleTime=-1  LimitOutput=on  UpperSaturationLimit=5  LowerSaturationLimit=-5  ICPrevOutput=DiscIntNeverNeededParam  ICPrevScaledInput=DiscIntNeverNeededParam
  Discrete-Time Integrator6 : DiscreteIntegrator  SampleTime=-1  LimitOutput=on  UpperSaturationLimit=0.4  LowerSaturationLimit=-0.4  ICPrevOutput=DiscIntNeverNeededParam  ICPrevScaledInput=DiscIntNeverNeededParam
  Discrete-Time Integrator7 : DiscreteIntegrator  SampleTime=-1  LimitOutput=on  UpperSaturationLimit=2  LowerSaturationLimit=-2  ICPrevOutput=DiscIntNeverNeededParam  ICPrevScaledInput=DiscIntNeverNeededParam
  Gain : Gain  Gain=0.77
  Gain1 : Gain  Gain=0.6
  Gain3 : Gain  Gain=-1
  MATLAB Function : MATLAB Function  TreatAsAtomicUnit=on
  MATLAB Function1 : MATLAB Function  TreatAsAtomicUnit=on
  MATLAB Function3 : MATLAB Function  TreatAsAtomicUnit=on
  MATLAB Function5 : MATLAB Function  TreatAsAtomicUnit=on
  Memory1 : Memory  InitialCondition=1
  Memory{2..4,6..8} (6 alike) : Memory
  Memory5 : Memory  InitialCondition=[0 0 0]'
  Saturation : Saturate  UpperLimit=1  LowerLimit=-1
  Scope1 : Scope
  Switch : Switch  Threshold=150  SaturateOnIntegerOverflow=off  InputSameDT=off
  To Workspace1 : ToWorkspace  VariableName=evsy6  SampleTime=-1
  event_1 : MATLAB Function  TreatAsAtomicUnit=on
  event_x2 : MATLAB Function  TreatAsAtomicUnit=on
  memory_1 : MATLAB Function  TreatAsAtomicUnit=on
  U_ipos : Outport  VectorParamsAs1DForOutWhenUnconnected=off
  U_iyaw : Outport  Port=2  VectorParamsAs1DForOutWhenUnconnected=off
  tag scope: e_yaw6=global
  wires:
  ref/1 -> Bus Selector/1
  state/1 -> Bus Selector1/1
  Bus Selector/1 -> Demux5/1  "<xi_d>"
  statej/1 -> Bus Selector2/1
  Bus Selector2/1 -> Demux1/1  "<xyz>"
  Demux1/1 -> MATLAB Function/4(xj)
  Demux1/2 -> MATLAB Function/5(yj)
  Discrete-Time Integrator1/1 -> MATLAB Function1/3(phiAlpha_int)
  statek/1 -> Bus Selector3/1
  Demux3/1 -> MATLAB Function/7(xk)
  Demux3/2 -> MATLAB Function/8(yk)
  Bus Selector3/1 -> Demux3/1  "<xyz>"
  MATLAB Function/1(phiAlpha) -> Gain3/1
  Demux3/3 -> MATLAB Function/9(zk)
  Demux1/3 -> MATLAB Function/6(zj)
  statel/1 -> Bus Selector4/1
  Demux7/1 -> MATLAB Function/10(xl)
  Demux7/2 -> MATLAB Function/11(yl)
  Demux7/3 -> MATLAB Function/12(zl)
  Bus Selector4/1 -> Demux7/1  "<xyz>"
  Bus Selector1/2 -> [YAW]  "<YAW>"
  [YAW] -> MATLAB Function1/5(yaw)
  MATLAB Function1/2(ui_yaw) -> U_iyaw/1
  MATLAB Function1/3(eyaw2) -> Memory1/1, Discrete-Time Integrator3/1
  Discrete-Time Integrator3/1 -> MATLAB Function1/6(ieyaw)
  [K_alpha] -> MATLAB Function1/7(KP)
  [params] -> MATLAB Function/25(params)
  statem/1 -> Bus Selector5/1
  Bus Selector5/1 -> Demux2/1  "<xyz>"
  Demux2/1 -> MATLAB Function/13(xm)
  Demux2/2 -> MATLAB Function/14(ym)
  Demux2/3 -> MATLAB Function/15(zm)
  Memory1/1 -> [e_yaw6]
  [e_yaw1] -> MATLAB Function1/8(eyaw1)
  [e_yaw3] -> MATLAB Function1/10(eyaw3)
  [e_yaw4] -> MATLAB Function1/11(eyaw4)
  [e_yaw2] -> MATLAB Function1/9("eyaw2 ")
  Discrete-Time Integrator4/1 -> MATLAB Function5/3(q_hat)
  Discrete-Time Integrator5/1 -> Saturation/1, MATLAB Function5/4(eta1)
  [L_obs] -> MATLAB Function5/1(L)
  MATLAB Function5/1(dot_hat_q) -> Discrete-Time Integrator4/1
  MATLAB Function1/1(Ui_pos) -> MATLAB Function5/6(u), U_ipos/1
  Bus Selector1/1 -> Demux4/1, MATLAB Function5/2(q)  "<xyz>"
  MATLAB Function5/2(dot_eta) -> Discrete-Time Integrator5/1
  Discrete-Time Integrator6/1 -> MATLAB Function5/5(eta2)
  MATLAB Function5/3(ddot_eta) -> Discrete-Time Integrator6/1
  staten/1 -> Bus Selector6/1
  Demux6/1 -> MATLAB Function/16(xn)
  Demux6/2 -> MATLAB Function/17(yn)
  Demux6/3 -> MATLAB Function/18(zn)
  Bus Selector6/1 -> Demux6/1  "<xyz>"
  [e_yaw5] -> MATLAB Function1/12(eyaw5)
  staten1/1 -> Bus Selector7/1
  Demux8/1 -> MATLAB Function/19(xo)
  Demux8/2 -> MATLAB Function/20(yo)
  Demux8/3 -> MATLAB Function/21(zo)
  Bus Selector7/1 -> Demux8/1  "<xyz>"
  [e_yaw7] -> MATLAB Function1/13(eyaw7)
  staten2/1 -> Bus Selector8/1
  Demux9/2 -> MATLAB Function/23(yp)
  Demux9/1 -> MATLAB Function/22(xp)
  Demux9/3 -> MATLAB Function/24(zp)
  Bus Selector8/1 -> Demux9/1  "<xyz>"
  [e_yaw8] -> MATLAB Function1/14(eyaw8)
  Bus Selector9/1 -> Demux10/1  "<xyz>"
  ref1/1 -> Bus Selector9/1
  Switch/1 -> MATLAB Function1/1(eta)
  Gain1/1 -> Switch/3
  Gain/1 -> Switch/1
  [gaz_time] -> Switch/2
  Saturation/1 -> Gain1/1, Gain/1
  ref2/1 -> Bus Selector10/1
  Bus Selector10/1 -> Demux11/1  "<xyz>"
  [x_sam] -> MATLAB Function3/2(xi)
  [z_sam] -> MATLAB Function3/4(zi)
  [y_sam] -> MATLAB Function3/3(yi)
  Memory2/1 -> memory_1/7("mx "), event_1/4(mx), [x_sam]
  Memory4/1 -> memory_1/9("mz "), event_1/6(mz), [z_sam]
  [norm_ey] -> MATLAB Function3/16(norm_ey)
  event_1/2(norm_ey) -> [norm_ey], memory_1/2(ey)
  memory_1/2(my) -> Memory3/1
  [norm_ex] -> MATLAB Function3/15(norm_ex)
  Memory5/1 -> MATLAB Function3/1(ui_prev)
  Demux4/2 -> memory_1/5(y), event_1/2(y), MATLAB Function/2(yi)
  Discrete-Time Integrator7/1 -> MATLAB Function3/14(iep)
  Demux4/3 -> memory_1/6(z), event_1/3(z), MATLAB Function/3(zi)
  MATLAB Function3/2(ep) -> Discrete-Time Integrator7/1
  MATLAB Function3/1(ui_gamma) -> MATLAB Function1/4(ui_gamma), Scope1/1, Memory5/1
  Demux4/1 -> MATLAB Function/1(xi), memory_1/4(x), event_1/1(x)
  [norm_ez] -> MATLAB Function3/17(norm_ez)
  memory_1/1(mx) -> Memory2/1
  event_1/1(norm_ex) -> [norm_ex], memory_1/1(ex)
  Memory3/1 -> [y_sam], memory_1/8("my "), event_1/5(my)
  event_1/3(norm_ez) -> [norm_ez], memory_1/3(ez)
  memory_1/3(mz) -> Memory4/1
  Demux10/1 -> MATLAB Function3/8(xr2)
  Demux11/1 -> MATLAB Function3/11(xr3)
  Demux5/1 -> MATLAB Function3/5(xr1)
  Demux10/2 -> MATLAB Function3/9(yr2)
  Demux11/2 -> MATLAB Function3/12(yr3)
  Demux5/2 -> MATLAB Function3/6(yr1)
  Demux10/3 -> MATLAB Function3/10(zr2)
  Demux11/3 -> MATLAB Function3/13(zr3)
  Demux5/3 -> MATLAB Function3/7(zr1)
  [K_con] -> MATLAB Function3/18(K_cts)
  [C0] -> event_1/7(c0)
  Gain3/1 -> MATLAB Function1/2(phiAlpha), Discrete-Time Integrator1/1
  Memory7/1 -> event_x2/6("i3 ")
  [norm_ez] -> event_x2/3(e3)
  [norm_ex] -> event_x2/1(e1)
  event_x2/2(i2) -> Memory8/1
  Memory8/1 -> To Workspace1/1, event_x2/5("i2 ")
  event_x2/1(i1) -> Memory6/1
  Memory6/1 -> event_x2/4("i1 ")
  event_x2/3(i3) -> Memory7/1
  [norm_ey] -> event_x2/2(e2)

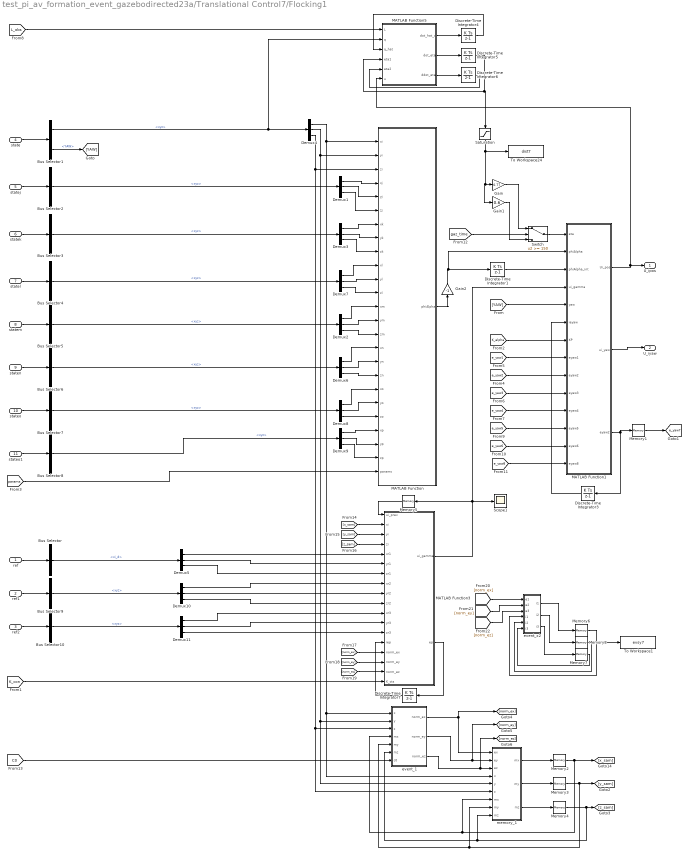
== system test_pi_av_formation_event_gazebodirected23a/Translational Control7/Flocking1 ==
  ref : Inport
  ref1 : Inport  Port=2
  ref2 : Inport  Port=3
  state : Inport  Port=4
  statej : Inport  Port=5
  statek : Inport  Port=6
  statel : Inport  Port=7
  statem : Inport  Port=8
  staten : Inport  Port=9
  stateo : Inport  Port=10
  stateo1 : Inport  Port=11
  Bus Selector : BusSelector  OutputSignals=xi_d
  Bus Selector1 : BusSelector  OutputSignals=xyz,YAW
  Bus Selector{2..10} (9 alike) : BusSelector  OutputSignals=xyz
  Demux{1..11} (11 alike) : Demux  Outputs=3
  Discrete-Time Integrator1 : DiscreteIntegrator  SampleTime=-1  LimitOutput=on  UpperSaturationLimit=2  LowerSaturationLimit=-2  ICPrevOutput=DiscIntNeverNeededParam  ICPrevScaledInput=DiscIntNeverNeededParam
  Discrete-Time Integrator3 : DiscreteIntegrator  SampleTime=-1  LimitOutput=on  UpperSaturationLimit=1  LowerSaturationLimit=-1  ICPrevOutput=DiscIntNeverNeededParam  ICPrevScaledInput=DiscIntNeverNeededParam
  Discrete-Time Integrator4 : DiscreteIntegrator  SampleTime=-1  LimitOutput=on  UpperSaturationLimit=5  LowerSaturationLimit=-5  ICPrevOutput=DiscIntNeverNeededParam  ICPrevScaledInput=DiscIntNeverNeededParam
  Discrete-Time Integrator5 : DiscreteIntegrator  SampleTime=-1  LimitOutput=on  UpperSaturationLimit=5  LowerSaturationLimit=-5  ICPrevOutput=DiscIntNeverNeededParam  ICPrevScaledInput=DiscIntNeverNeededParam
  Discrete-Time Integrator6 : DiscreteIntegrator  SampleTime=-1  LimitOutput=on  UpperSaturationLimit=0.4  LowerSaturationLimit=-0.4  ICPrevOutput=DiscIntNeverNeededParam  ICPrevScaledInput=DiscIntNeverNeededParam
  Discrete-Time Integrator7 : DiscreteIntegrator  SampleTime=-1  LimitOutput=on  UpperSaturationLimit=2  LowerSaturationLimit=-2  ICPrevOutput=DiscIntNeverNeededParam  ICPrevScaledInput=DiscIntNeverNeededParam
  Gain : Gain  Gain=0.77
  Gain1 : Gain  Gain=0.6
  Gain2 : Gain  Gain=-1
  MATLAB Function : MATLAB Function  TreatAsAtomicUnit=on
  MATLAB Function1 : MATLAB Function  TreatAsAtomicUnit=on
  MATLAB Function3 : MATLAB Function  TreatAsAtomicUnit=on
  MATLAB Function5 : MATLAB Function  TreatAsAtomicUnit=on
  Memory1 : Memory  InitialCondition=1
  Memory{2..4,6..8} (6 alike) : Memory
  Memory5 : Memory  InitialCondition=[0 0 0]'
  Saturation : Saturate  UpperLimit=1  LowerLimit=-1
  Scope1 : Scope
  Switch : Switch  Threshold=150  SaturateOnIntegerOverflow=off  InputSameDT=off
  To Workspace1 : ToWorkspace  VariableName=evsy7  SampleTime=-1
  To Workspace24 : ToWorkspace  VariableName=dist7  SampleTime=-1
  event_1 : MATLAB Function  TreatAsAtomicUnit=on
  event_x2 : MATLAB Function  TreatAsAtomicUnit=on
  memory_1 : MATLAB Function  TreatAsAtomicUnit=on
  U_ipos : Outport  VectorParamsAs1DForOutWhenUnconnected=off
  U_iyaw : Outport  Port=2  VectorParamsAs1DForOutWhenUnconnected=off
  tag scope: e_yaw7=global
  wires:
  [e_yaw6] -> MATLAB Function1/13(eyaw6)
  Bus Selector7/1 -> Demux8/1  "<xyz>"
  Demux8/3 -> MATLAB Function/21(zo)
  Demux8/2 -> MATLAB Function/20(yo)
  Demux8/1 -> MATLAB Function/19(xo)
  stateo/1 -> Bus Selector7/1
  [e_yaw5] -> MATLAB Function1/12(eyaw5)
  Bus Selector6/1 -> Demux6/1  "<xyz>"
  Demux6/3 -> MATLAB Function/18(zn)
  Demux6/2 -> MATLAB Function/17(yn)
  Demux6/1 -> MATLAB Function/16(xn)
  staten/1 -> Bus Selector6/1
  MATLAB Function5/3(ddot_eta) -> Discrete-Time Integrator6/1
  Discrete-Time Integrator6/1 -> MATLAB Function5/5(eta2)
  MATLAB Function5/2(dot_eta) -> Discrete-Time Integrator5/1
  Bus Selector1/1 -> Demux4/1, MATLAB Function5/2(q)  "<xyz>"
  MATLAB Function1/1(Ui_pos) -> U_ipos/1, MATLAB Function5/6(u)
  MATLAB Function5/1(dot_hat_q) -> Discrete-Time Integrator4/1
  [L_obs] -> MATLAB Function5/1(L)
  Discrete-Time Integrator5/1 -> MATLAB Function5/4(eta1), Saturation/1
  Discrete-Time Integrator4/1 -> MATLAB Function5/3(q_hat)
  [e_yaw2] -> MATLAB Function1/9("eyaw2 ")
  [e_yaw4] -> MATLAB Function1/11(eyaw4)
  [e_yaw3] -> MATLAB Function1/10(eyaw3)
  [e_yaw1] -> MATLAB Function1/8(eyaw1)
  Memory1/1 -> [e_yaw7]
  Demux2/3 -> MATLAB Function/15(zm)
  Demux2/2 -> MATLAB Function/14(ym)
  Demux2/1 -> MATLAB Function/13(xm)
  Bus Selector5/1 -> Demux2/1  "<xyz>"
  statem/1 -> Bus Selector5/1
  [params] -> MATLAB Function/25(params)
  [K_alpha] -> MATLAB Function1/7(KP)
  Discrete-Time Integrator3/1 -> MATLAB Function1/6(ieyaw)
  MATLAB Function1/3(eyaw2) -> Memory1/1, Discrete-Time Integrator3/1
  MATLAB Function1/2(ui_yaw) -> U_iyaw/1
  [YAW] -> MATLAB Function1/5(yaw)
  Bus Selector1/2 -> [YAW]  "<YAW>"
  Bus Selector4/1 -> Demux7/1  "<xyz>"
  Demux7/3 -> MATLAB Function/12(zl)
  Demux7/2 -> MATLAB Function/11(yl)
  Demux7/1 -> MATLAB Function/10(xl)
  statel/1 -> Bus Selector4/1
  Demux1/3 -> MATLAB Function/6(zj)
  Demux3/3 -> MATLAB Function/9(zk)
  Demux4/3 -> memory_1/6(z), event_1/3(z), MATLAB Function/3(zi)
  MATLAB Function/1(phiAlpha) -> Gain2/1
  Bus Selector3/1 -> Demux3/1  "<xyz>"
  Demux3/2 -> MATLAB Function/8(yk)
  Demux3/1 -> MATLAB Function/7(xk)
  statek/1 -> Bus Selector3/1
  Discrete-Time Integrator1/1 -> MATLAB Function1/3(phiAlpha_int)
  Demux1/2 -> MATLAB Function/5(yj)
  Demux1/1 -> MATLAB Function/4(xj)
  Demux4/2 -> memory_1/5(y), event_1/2(y), MATLAB Function/2(yi)
  Demux4/1 -> memory_1/4(x), event_1/1(x), MATLAB Function/1(xi)
  Bus Selector2/1 -> Demux1/1  "<xyz>"
  statej/1 -> Bus Selector2/1
  Bus Selector/1 -> Demux5/1  "<xi_d>"
  state/1 -> Bus Selector1/1
  ref/1 -> Bus Selector/1
  stateo1/1 -> Bus Selector8/1
  Demux9/2 -> MATLAB Function/23(yp)
  Demux9/1 -> MATLAB Function/22(xp)
  Demux9/3 -> MATLAB Function/24(zp)
  Bus Selector8/1 -> Demux9/1  "<xyz>"
  [e_yaw8] -> MATLAB Function1/14(eyaw8)
  ref1/1 -> Bus Selector9/1
  Bus Selector9/1 -> Demux10/1  "<xyz>"
  Bus Selector10/1 -> Demux11/1  "<xyz>"
  ref2/1 -> Bus Selector10/1
  Saturation/1 -> To Workspace24/1, Gain1/1, Gain/1
  Switch/1 -> MATLAB Function1/1(eta)
  Gain1/1 -> Switch/3
  Gain/1 -> Switch/1
  [gaz_time] -> Switch/2
  memory_1/1(mx) -> Memory2/1
  Memory5/1 -> MATLAB Function3/1(ui_prev)
  memory_1/2(my) -> Memory3/1
  [norm_ez] -> MATLAB Function3/17(norm_ez)
  Discrete-Time Integrator7/1 -> MATLAB Function3/14(iep)
  Memory4/1 -> memory_1/9("mz "), event_1/6(mz), [z_sam]
  [norm_ex] -> MATLAB Function3/15(norm_ex)
  event_1/3(norm_ez) -> [norm_ez], memory_1/3(ez)
  event_1/2(norm_ey) -> [norm_ey], memory_1/2(ey)
  [x_sam] -> MATLAB Function3/2(xi)
  Memory2/1 -> memory_1/7("mx "), event_1/4(mx), [x_sam]
  [z_sam] -> MATLAB Function3/4(zi)
  [norm_ey] -> MATLAB Function3/16(norm_ey)
  Memory3/1 -> [y_sam], memory_1/8("my "), event_1/5(my)
  [y_sam] -> MATLAB Function3/3(yi)
  memory_1/3(mz) -> Memory4/1
  MATLAB Function3/1(ui_gamma) -> MATLAB Function1/4(ui_gamma), Scope1/1, Memory5/1
  event_1/1(norm_ex) -> [norm_ex], memory_1/1(ex)
  MATLAB Function3/2(ep) -> Discrete-Time Integrator7/1
  Demux11/1 -> MATLAB Function3/11(xr3)
  Demux10/1 -> MATLAB Function3/8(xr2)
  Demux11/2 -> MATLAB Function3/12(yr3)
  Demux5/1 -> MATLAB Function3/5(xr1)
  Demux10/2 -> MATLAB Function3/9(yr2)
  Demux11/3 -> MATLAB Function3/13(zr3)
  Demux5/2 -> MATLAB Function3/6(yr1)
  Demux10/3 -> MATLAB Function3/10(zr2)
  Demux5/3 -> MATLAB Function3/7(zr1)
  [K_con] -> MATLAB Function3/18(K_cts)
  [C0] -> event_1/7(c0)
  Gain2/1 -> Discrete-Time Integrator1/1, MATLAB Function1/2(phiAlpha)
  Memory7/1 -> event_x2/6("i3 ")
  [norm_ez] -> event_x2/3(e3)
  [norm_ex] -> event_x2/1(e1)
  event_x2/2(i2) -> Memory8/1
  Memory8/1 -> To Workspace1/1, event_x2/5("i2 ")
  event_x2/1(i1) -> Memory6/1
  Memory6/1 -> event_x2/4("i1 ")
  event_x2/3(i3) -> Memory7/1
  [norm_ey] -> event_x2/2(e2)
